simulink model "Diagrama de Dron NERV Protocol"  (R2026a)
settings: Solver=VariableStepAuto
undefined symbols (not defined in the file): A, adelante, antihorario, atras, bajar, boton1, boton2, boton3, boton4, boton5, camara, controladorm, derecha, encendido, G, gantihorario, ghorario, horario, izquierda, joystick1, joystick2, microcontrolador, modulowifi, S, subir, video

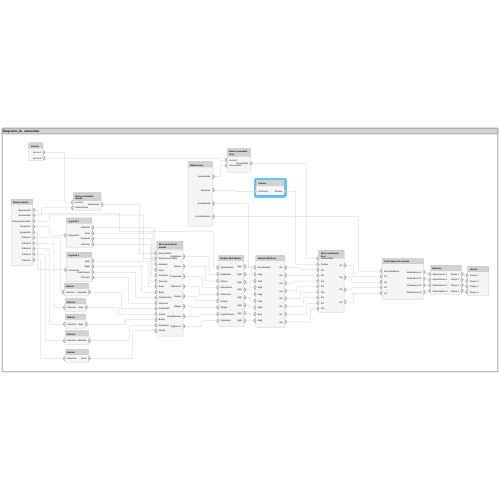
[thumbnail: Simulink's stored preview of the top-level diagram]
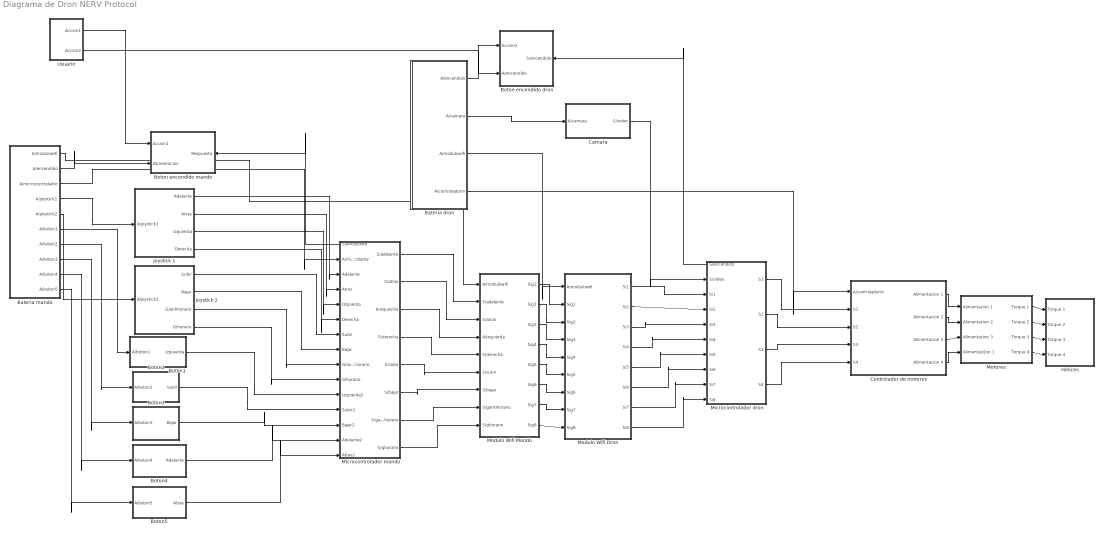
== system Diagrama de Dron NERV Protocol ==
  Bateria dron : Subsystem
      settings: PortSchema="{\"entries\":[{\"content\":{\"headerSize\":26,\"margin\":15,\"minimumSpacing\":25,\"sides\":[{\"content\":{},\"type\":\"ConnectorPlacement.EquallySpacedRectSide\",\"uuid\":\"2bf6d042-84ef-4730-88f6-3dff55cafecf\"},{\"content\":{\"connectorIds\":[\"Out1\",\"Out2\",\"Out3\",\"Out4\"],\"side\":\"RIGHT\"},\"type\":\"ConnectorPlacement.EquallySpacedRectSide\",\"uuid\":\"8f67bf94-d3d5-4da5-abec-0099f91d79d4\"},{\"content\":{\"side\":\"TOP\"},\"type\":\"ConnectorPlacement.EquallySpacedRectSide\",\"uuid\":\"7fdef67b-3e3b-4487-991c-040d13a0e676\"}]},\"type\":\"ConnectorPlacement.EquallySpacedConnector\",\"uuid\":\"d2ee6619-957d-4521-bbff-daa84c43e1b5\"}],\"packageUris\":[\"http://schema.mathworks.com/mf0/Connector/R2020b\"],\"version\":\"1.0\"}"
  Bateria mando : Subsystem
      settings: PortSchema="{\"entries\":[{\"content\":{\"headerSize\":26,\"margin\":15,\"minimumSpacing\":25,\"sides\":[{\"content\":{},\"type\":\"ConnectorPlacement.EquallySpacedRectSide\",\"uuid\":\"c8c9d0d9-9f51-4378-b4f1-417ae5560a64\"},{\"content\":{\"connectorIds\":[\"Out1\",\"Out2\",\"Out3\",\"Out4\",\"Out5\",\"Out6\",\"Out7\",\"Out8\",\"Out9\",\"Out10\"],\"side\":\"RIGHT\"},\"type\":\"ConnectorPlacement.EquallySpacedRectSide\",\"uuid\":\"af341b24-fdfa-4fbe-98c5-0f07d2be8a36\"},{\"content\":{\"side\":\"TOP\"},\"type\":\"ConnectorPlacement.EquallySpacedRectSide\",\"uuid\":\"c7c4f077-f713-4504-becb-cb3de254be2a\"}]},\"type\":\"ConnectorPlacement.EquallySpacedConnector\",\"uuid\":\"2a74e7c1-b664-434d-aa05-bb22f18d4dbf\"}],\"packageUris\":[\"http://schema.mathworks.com/mf0/Connector/R2020b\"],\"version\":\"1.0\"}"
  Boton encendido dron : Subsystem
      settings: PortSchema="{\"entries\":[{\"content\":{\"headerSize\":26,\"margin\":15,\"minimumSpacing\":25,\"sides\":[{\"content\":{\"connectorIds\":[\"In1\",\"In2\"]},\"type\":\"ConnectorPlacement.EquallySpacedRectSide\",\"uuid\":\"c8c9d0d9-9f51-4378-b4f1-417ae5560a64\"},{\"content\":{\"connectorIds\":[\"In3\"],\"side\":\"RIGHT\"},\"type\":\"ConnectorPlacement.EquallySpacedRectSide\",\"uuid\":\"af341b24-fdfa-4fbe-98c5-0f07d2be8a36\"},{\"content\":{\"side\":\"TOP\"},\"type\":\"ConnectorPlacement.EquallySpacedRectSide\",\"uuid\":\"c7c4f077-f713-4504-becb-cb3de254be2a\"}]},\"type\":\"ConnectorPlacement.EquallySpacedConnector\",\"uuid\":\"2a74e7c1-b664-434d-aa05-bb22f18d4dbf\"}],\"packageUris\":[\"http://schema.mathworks.com/mf0/Connector/R2020b\"],\"version\":\"1.0\"}"
  Boton encendido mando : Subsystem
      settings: PortSchema="{\"entries\":[{\"content\":{\"headerSize\":26,\"margin\":15,\"minimumSpacing\":25,\"sides\":[{\"content\":{\"connectorIds\":[\"In1\",\"In2\"]},\"type\":\"ConnectorPlacement.EquallySpacedRectSide\",\"uuid\":\"c8c9d0d9-9f51-4378-b4f1-417ae5560a64\"},{\"content\":{\"connectorIds\":[\"In3\"],\"side\":\"RIGHT\"},\"type\":\"ConnectorPlacement.EquallySpacedRectSide\",\"uuid\":\"af341b24-fdfa-4fbe-98c5-0f07d2be8a36\"},{\"content\":{\"side\":\"TOP\"},\"type\":\"ConnectorPlacement.EquallySpacedRectSide\",\"uuid\":\"c7c4f077-f713-4504-becb-cb3de254be2a\"}]},\"type\":\"ConnectorPlacement.EquallySpacedConnector\",\"uuid\":\"2a74e7c1-b664-434d-aa05-bb22f18d4dbf\"}],\"packageUris\":[\"http://schema.mathworks.com/mf0/Connector/R2020b\"],\"version\":\"1.0\"}"
  Boton1 : Subsystem
      settings: PortSchema="{\"entries\":[{\"content\":{\"headerSize\":26,\"margin\":15,\"minimumSpacing\":25,\"sides\":[{\"content\":{\"connectorIds\":[\"In1\"]},\"type\":\"ConnectorPlacement.EquallySpacedRectSide\",\"uuid\":\"859b65f9-1e56-49db-ad0e-625ee06f8163\"},{\"content\":{\"connectorIds\":[\"Out1\"],\"side\":\"RIGHT\"},\"type\":\"ConnectorPlacement.EquallySpacedRectSide\",\"uuid\":\"c49bccff-8b78-479d-ba62-905aef2a1b5e\"},{\"content\":{\"side\":\"TOP\"},\"type\":\"ConnectorPlacement.EquallySpacedRectSide\",\"uuid\":\"337def3d-9fc7-40b9-833c-a49097c9210f\"}]},\"type\":\"ConnectorPlacement.EquallySpacedConnector\",\"uuid\":\"a8accb01-4db9-4c00-8da7-dedce669f5d7\"}],\"packageUris\":[\"http://schema.mathworks.com/mf0/Connector/R2020b\"],\"version\":\"1.0\"}"
  Boton2 : Subsystem
      settings: PortSchema="{\"entries\":[{\"content\":{\"headerSize\":26,\"margin\":15,\"minimumSpacing\":25,\"sides\":[{\"content\":{\"connectorIds\":[\"In1\"]},\"type\":\"ConnectorPlacement.EquallySpacedRectSide\",\"uuid\":\"859b65f9-1e56-49db-ad0e-625ee06f8163\"},{\"content\":{\"connectorIds\":[\"Out1\"],\"side\":\"RIGHT\"},\"type\":\"ConnectorPlacement.EquallySpacedRectSide\",\"uuid\":\"c49bccff-8b78-479d-ba62-905aef2a1b5e\"},{\"content\":{\"side\":\"TOP\"},\"type\":\"ConnectorPlacement.EquallySpacedRectSide\",\"uuid\":\"337def3d-9fc7-40b9-833c-a49097c9210f\"}]},\"type\":\"ConnectorPlacement.EquallySpacedConnector\",\"uuid\":\"a8accb01-4db9-4c00-8da7-dedce669f5d7\"}],\"packageUris\":[\"http://schema.mathworks.com/mf0/Connector/R2020b\"],\"version\":\"1.0\"}"
  Boton3 : Subsystem
      settings: PortSchema="{\"entries\":[{\"content\":{\"headerSize\":26,\"margin\":15,\"minimumSpacing\":25,\"sides\":[{\"content\":{\"connectorIds\":[\"In1\"]},\"type\":\"ConnectorPlacement.EquallySpacedRectSide\",\"uuid\":\"859b65f9-1e56-49db-ad0e-625ee06f8163\"},{\"content\":{\"connectorIds\":[\"Out1\"],\"side\":\"RIGHT\"},\"type\":\"ConnectorPlacement.EquallySpacedRectSide\",\"uuid\":\"c49bccff-8b78-479d-ba62-905aef2a1b5e\"},{\"content\":{\"side\":\"TOP\"},\"type\":\"ConnectorPlacement.EquallySpacedRectSide\",\"uuid\":\"337def3d-9fc7-40b9-833c-a49097c9210f\"}]},\"type\":\"ConnectorPlacement.EquallySpacedConnector\",\"uuid\":\"a8accb01-4db9-4c00-8da7-dedce669f5d7\"}],\"packageUris\":[\"http://schema.mathworks.com/mf0/Connector/R2020b\"],\"version\":\"1.0\"}"
  Boton4 : Subsystem
      settings: PortSchema="{\"entries\":[{\"content\":{\"headerSize\":26,\"margin\":15,\"minimumSpacing\":25,\"sides\":[{\"content\":{\"connectorIds\":[\"In1\"]},\"type\":\"ConnectorPlacement.EquallySpacedRectSide\",\"uuid\":\"859b65f9-1e56-49db-ad0e-625ee06f8163\"},{\"content\":{\"connectorIds\":[\"Out1\"],\"side\":\"RIGHT\"},\"type\":\"ConnectorPlacement.EquallySpacedRectSide\",\"uuid\":\"c49bccff-8b78-479d-ba62-905aef2a1b5e\"},{\"content\":{\"side\":\"TOP\"},\"type\":\"ConnectorPlacement.EquallySpacedRectSide\",\"uuid\":\"337def3d-9fc7-40b9-833c-a49097c9210f\"}]},\"type\":\"ConnectorPlacement.EquallySpacedConnector\",\"uuid\":\"a8accb01-4db9-4c00-8da7-dedce669f5d7\"}],\"packageUris\":[\"http://schema.mathworks.com/mf0/Connector/R2020b\"],\"version\":\"1.0\"}"
  Boton5 : Subsystem
      settings: PortSchema="{\"entries\":[{\"content\":{\"headerSize\":26,\"margin\":15,\"minimumSpacing\":25,\"sides\":[{\"content\":{\"connectorIds\":[\"In1\"]},\"type\":\"ConnectorPlacement.EquallySpacedRectSide\",\"uuid\":\"859b65f9-1e56-49db-ad0e-625ee06f8163\"},{\"content\":{\"connectorIds\":[\"Out1\"],\"side\":\"RIGHT\"},\"type\":\"ConnectorPlacement.EquallySpacedRectSide\",\"uuid\":\"c49bccff-8b78-479d-ba62-905aef2a1b5e\"},{\"content\":{\"side\":\"TOP\"},\"type\":\"ConnectorPlacement.EquallySpacedRectSide\",\"uuid\":\"337def3d-9fc7-40b9-833c-a49097c9210f\"}]},\"type\":\"ConnectorPlacement.EquallySpacedConnector\",\"uuid\":\"a8accb01-4db9-4c00-8da7-dedce669f5d7\"}],\"packageUris\":[\"http://schema.mathworks.com/mf0/Connector/R2020b\"],\"version\":\"1.0\"}"
  Camara : Subsystem
      settings: PortSchema="{\"entries\":[{\"content\":{\"headerSize\":26,\"margin\":15,\"minimumSpacing\":25,\"sides\":[{\"content\":{\"connectorIds\":[\"In1\"]},\"type\":\"ConnectorPlacement.EquallySpacedRectSide\",\"uuid\":\"879727f6-324c-4f5e-9dc1-ac479d9c48af\"},{\"content\":{\"connectorIds\":[\"Out1\"],\"side\":\"RIGHT\"},\"type\":\"ConnectorPlacement.EquallySpacedRectSide\",\"uuid\":\"f3855134-d9a3-4d8c-bf73-dc4ed9d71427\"},{\"content\":{\"side\":\"TOP\"},\"type\":\"ConnectorPlacement.EquallySpacedRectSide\",\"uuid\":\"f26ad25d-e4a2-425b-a9d5-96d823958aa9\"}]},\"type\":\"ConnectorPlacement.EquallySpacedConnector\",\"uuid\":\"a98458b0-d022-4598-9285-5429fabca4b2\"}],\"packageUris\":[\"http://schema.mathworks.com/mf0/Connector/R2020b\"],\"version\":\"1.0\"}"
  Controlador de motores : Subsystem
      settings: PortSchema="{\"entries\":[{\"content\":{\"headerSize\":26,\"margin\":15,\"minimumSpacing\":25,\"sides\":[{\"content\":{\"connectorIds\":[\"In3\",\"In4\",\"In5\",\"In1\",\"In2\"]},\"type\":\"ConnectorPlacement.EquallySpacedRectSide\",\"uuid\":\"2bf6d042-84ef-4730-88f6-3dff55cafecf\"},{\"content\":{\"connectorIds\":[\"Out1\",\"Out2\",\"Out3\",\"Out4\"],\"side\":\"RIGHT\"},\"type\":\"ConnectorPlacement.EquallySpacedRectSide\",\"uuid\":\"8f67bf94-d3d5-4da5-abec-0099f91d79d4\"},{\"content\":{\"side\":\"TOP\"},\"type\":\"ConnectorPlacement.EquallySpacedRectSide\",\"uuid\":\"7fdef67b-3e3b-4487-991c-040d13a0e676\"},{\"content\":{\"side\":\"BOTTOM\"},\"type\":\"ConnectorPlacement.EquallySpacedRectSide\",\"uuid\":\"0c2c01ed-c52d-4b0b-a737-70a441f21ba4\"}]},\"type\":\"ConnectorPlacement.EquallySpacedConnector\",\"uuid\":\"d2ee6619-957d-4521-bbff-daa84c43e1b5\"}],\"packageUris\":[\"http://schema.mathworks.com/mf0/Connector/R2020b\"],\"version\":\"1.0\"}"
  Helices : Subsystem
      settings: PortSchema="{\"entries\":[{\"content\":{\"headerSize\":26,\"margin\":15,\"minimumSpacing\":25,\"sides\":[{\"content\":{\"connectorIds\":[\"In1\",\"In2\",\"In3\",\"In4\"]},\"type\":\"ConnectorPlacement.EquallySpacedRectSide\",\"uuid\":\"2bf6d042-84ef-4730-88f6-3dff55cafecf\"},{\"content\":{\"side\":\"RIGHT\"},\"type\":\"ConnectorPlacement.EquallySpacedRectSide\",\"uuid\":\"8f67bf94-d3d5-4da5-abec-0099f91d79d4\"},{\"content\":{\"side\":\"TOP\"},\"type\":\"ConnectorPlacement.EquallySpacedRectSide\",\"uuid\":\"7fdef67b-3e3b-4487-991c-040d13a0e676\"}]},\"type\":\"ConnectorPlacement.EquallySpacedConnector\",\"uuid\":\"d2ee6619-957d-4521-bbff-daa84c43e1b5\"}],\"packageUris\":[\"http://schema.mathworks.com/mf0/Connector/R2020b\"],\"version\":\"1.0\"}"
  Joystick 1 : Subsystem
      settings: PortSchema="{\"entries\":[{\"content\":{\"headerSize\":26,\"margin\":15,\"minimumSpacing\":25,\"sides\":[{\"content\":{\"connectorIds\":[\"In1\"]},\"type\":\"ConnectorPlacement.EquallySpacedRectSide\",\"uuid\":\"2bf6d042-84ef-4730-88f6-3dff55cafecf\"},{\"content\":{\"connectorIds\":[\"Out1\",\"Out2\",\"Out3\",\"Out4\"],\"side\":\"RIGHT\"},\"type\":\"ConnectorPlacement.EquallySpacedRectSide\",\"uuid\":\"8f67bf94-d3d5-4da5-abec-0099f91d79d4\"},{\"content\":{\"side\":\"TOP\"},\"type\":\"ConnectorPlacement.EquallySpacedRectSide\",\"uuid\":\"7fdef67b-3e3b-4487-991c-040d13a0e676\"}]},\"type\":\"ConnectorPlacement.EquallySpacedConnector\",\"uuid\":\"d2ee6619-957d-4521-bbff-daa84c43e1b5\"}],\"packageUris\":[\"http://schema.mathworks.com/mf0/Connector/R2020b\"],\"version\":\"1.0\"}"
  Joystick 2 : Subsystem
      settings: PortSchema="{\"entries\":[{\"content\":{\"headerSize\":26,\"margin\":15,\"minimumSpacing\":25,\"sides\":[{\"content\":{\"connectorIds\":[\"In1\"]},\"type\":\"ConnectorPlacement.EquallySpacedRectSide\",\"uuid\":\"2bf6d042-84ef-4730-88f6-3dff55cafecf\"},{\"content\":{\"connectorIds\":[\"Out1\",\"Out2\",\"Out3\",\"Out4\"],\"side\":\"RIGHT\"},\"type\":\"ConnectorPlacement.EquallySpacedRectSide\",\"uuid\":\"8f67bf94-d3d5-4da5-abec-0099f91d79d4\"},{\"content\":{\"side\":\"TOP\"},\"type\":\"ConnectorPlacement.EquallySpacedRectSide\",\"uuid\":\"7fdef67b-3e3b-4487-991c-040d13a0e676\"}]},\"type\":\"ConnectorPlacement.EquallySpacedConnector\",\"uuid\":\"d2ee6619-957d-4521-bbff-daa84c43e1b5\"}],\"packageUris\":[\"http://schema.mathworks.com/mf0/Connector/R2020b\"],\"version\":\"1.0\"}"
  Microcontrolador dron : Subsystem
      settings: PortSchema="{\"entries\":[{\"content\":{\"headerSize\":26,\"margin\":15,\"minimumSpacing\":25,\"sides\":[{\"content\":{\"connectorIds\":[\"Out5\",\"In1\",\"In2\",\"In3\",\"In4\",\"In5\",\"In6\",\"In7\",\"In8\",\"In9\"]},\"type\":\"ConnectorPlacement.EquallySpacedRectSide\",\"uuid\":\"859b65f9-1e56-49db-ad0e-625ee06f8163\"},{\"content\":{\"connectorIds\":[\"Out1\",\"Out2\",\"Out3\",\"Out4\"],\"side\":\"RIGHT\"},\"type\":\"ConnectorPlacement.EquallySpacedRectSide\",\"uuid\":\"c49bccff-8b78-479d-ba62-905aef2a1b5e\"},{\"content\":{\"side\":\"TOP\"},\"type\":\"ConnectorPlacement.EquallySpacedRectSide\",\"uuid\":\"337def3d-9fc7-40b9-833c-a49097c9210f\"}]},\"type\":\"ConnectorPlacement.EquallySpacedConnector\",\"uuid\":\"a8accb01-4db9-4c00-8da7-dedce669f5d7\"}],\"packageUris\":[\"http://schema.mathworks.com/mf0/Connector/R2020b\"],\"version\":\"1.0\"}"
  Microcontrolador mando : Subsystem
      settings: PortSchema="{\"entries\":[{\"content\":{\"headerSize\":26,\"margin\":15,\"minimumSpacing\":25,\"sides\":[{\"content\":{\"connectorIds\":[\"Out9\",\"In1\",\"In2\",\"In3\",\"In4\",\"In5\",\"In6\",\"In7\",\"In8\",\"In9\",\"In10\",\"In11\",\"In12\",\"In13\",\"In14\"]},\"type\":\"ConnectorPlacement.EquallySpacedRectSide\",\"uuid\":\"859b65f9-1e56-49db-ad0e-625ee06f8163\"},{\"content\":{\"connectorIds\":[\"Out1\",\"Out2\",\"Out3\",\"Out4\",\"Out5\",\"Out6\",\"Out7\",\"Out8\"],\"side\":\"RIGHT\"},\"type\":\"ConnectorPlacement.EquallySpacedRectSide\",\"uuid\":\"c49bccff-8b78-479d-ba62-905aef2a1b5e\"},{\"content\":{\"side\":\"TOP\"},\"type\":\"ConnectorPlacement.EquallySpacedRectSide\",\"uuid\":\"337def3d-9fc7-40b9-833c-a49097c9210f\"}]},\"type\":\"ConnectorPlacement.EquallySpacedConnector\",\"uuid\":\"a8accb01-4db9-4c00-8da7-dedce669f5d7\"}],\"packageUris\":[\"http://schema.mathworks.com/mf0/Connector/R2020b\"],\"version\":\"1.0\"}"
  Modulo Wifi Dron : Subsystem
      settings: PortSchema="{\"entries\":[{\"content\":{\"headerSize\":26,\"margin\":15,\"minimumSpacing\":25,\"sides\":[{\"content\":{\"connectorIds\":[\"In1\",\"In2\",\"In3\",\"In4\",\"In5\",\"In6\",\"In7\",\"In8\",\"In9\"]},\"type\":\"ConnectorPlacement.EquallySpacedRectSide\",\"uuid\":\"2bf6d042-84ef-4730-88f6-3dff55cafecf\"},{\"content\":{\"connectorIds\":[\"Out1\",\"Out2\",\"Out3\",\"Out4\",\"Out5\",\"Out6\",\"Out7\",\"Out8\"],\"side\":\"RIGHT\"},\"type\":\"ConnectorPlacement.EquallySpacedRectSide\",\"uuid\":\"8f67bf94-d3d5-4da5-abec-0099f91d79d4\"},{\"content\":{\"side\":\"TOP\"},\"type\":\"ConnectorPlacement.EquallySpacedRectSide\",\"uuid\":\"7fdef67b-3e3b-4487-991c-040d13a0e676\"}]},\"type\":\"ConnectorPlacement.EquallySpacedConnector\",\"uuid\":\"d2ee6619-957d-4521-bbff-daa84c43e1b5\"}],\"packageUris\":[\"http://schema.mathworks.com/mf0/Connector/R2020b\"],\"version\":\"1.0\"}"
  Modulo Wifi Mando : Subsystem
      settings: PortSchema="{\"entries\":[{\"content\":{\"headerSize\":26,\"margin\":15,\"minimumSpacing\":25,\"sides\":[{\"content\":{\"connectorIds\":[\"In1\",\"In2\",\"In3\",\"In4\",\"In5\",\"In6\",\"In7\",\"In8\",\"In9\"]},\"type\":\"ConnectorPlacement.EquallySpacedRectSide\",\"uuid\":\"2bf6d042-84ef-4730-88f6-3dff55cafecf\"},{\"content\":{\"connectorIds\":[\"Out1\",\"Out2\",\"Out3\",\"Out4\",\"Out5\",\"Out6\",\"Out7\",\"Out8\"],\"side\":\"RIGHT\"},\"type\":\"ConnectorPlacement.EquallySpacedRectSide\",\"uuid\":\"8f67bf94-d3d5-4da5-abec-0099f91d79d4\"},{\"content\":{\"side\":\"TOP\"},\"type\":\"ConnectorPlacement.EquallySpacedRectSide\",\"uuid\":\"7fdef67b-3e3b-4487-991c-040d13a0e676\"}]},\"type\":\"ConnectorPlacement.EquallySpacedConnector\",\"uuid\":\"d2ee6619-957d-4521-bbff-daa84c43e1b5\"}],\"packageUris\":[\"http://schema.mathworks.com/mf0/Connector/R2020b\"],\"version\":\"1.0\"}"
  Motores : Subsystem
      settings: PortSchema="{\"entries\":[{\"content\":{\"headerSize\":26,\"margin\":15,\"minimumSpacing\":25,\"sides\":[{\"content\":{\"connectorIds\":[\"In1\",\"In2\",\"In3\",\"In4\"]},\"type\":\"ConnectorPlacement.EquallySpacedRectSide\",\"uuid\":\"2bf6d042-84ef-4730-88f6-3dff55cafecf\"},{\"content\":{\"connectorIds\":[\"Out1\",\"Out2\",\"Out3\",\"Out4\"],\"side\":\"RIGHT\"},\"type\":\"ConnectorPlacement.EquallySpacedRectSide\",\"uuid\":\"8f67bf94-d3d5-4da5-abec-0099f91d79d4\"},{\"content\":{\"side\":\"TOP\"},\"type\":\"ConnectorPlacement.EquallySpacedRectSide\",\"uuid\":\"7fdef67b-3e3b-4487-991c-040d13a0e676\"}]},\"type\":\"ConnectorPlacement.EquallySpacedConnector\",\"uuid\":\"d2ee6619-957d-4521-bbff-daa84c43e1b5\"}],\"packageUris\":[\"http://schema.mathworks.com/mf0/Connector/R2020b\"],\"version\":\"1.0\"}"
  Usuario : Subsystem
      settings: PortSchema="{\"entries\":[{\"content\":{\"headerSize\":26,\"margin\":15,\"minimumSpacing\":25,\"sides\":[{\"content\":{},\"type\":\"ConnectorPlacement.EquallySpacedRectSide\",\"uuid\":\"c8c9d0d9-9f51-4378-b4f1-417ae5560a64\"},{\"content\":{\"connectorIds\":[\"Out1\",\"Out2\"],\"side\":\"RIGHT\"},\"type\":\"ConnectorPlacement.EquallySpacedRectSide\",\"uuid\":\"af341b24-fdfa-4fbe-98c5-0f07d2be8a36\"},{\"content\":{\"side\":\"TOP\"},\"type\":\"ConnectorPlacement.EquallySpacedRectSide\",\"uuid\":\"c7c4f077-f713-4504-becb-cb3de254be2a\"}]},\"type\":\"ConnectorPlacement.EquallySpacedConnector\",\"uuid\":\"2a74e7c1-b664-434d-aa05-bb22f18d4dbf\"}],\"packageUris\":[\"http://schema.mathworks.com/mf0/Connector/R2020b\"],\"version\":\"1.0\"}"
  wires:
  Motores/4(Torque 4) -> Helices/4(Torque 4)
  Motores/3(Torque 3) -> Helices/3(Torque 3)
  Motores/2(Torque 2) -> Helices/2(Torque 2)
  Motores/1(Torque 1) -> Helices/1(Torque 1)
  Controlador de motores/4(Alimentacion 4) -> Motores/4(Alimentaci[on 1)
  Controlador de motores/3(Alimentacion 3) -> Motores/3(Alimentacion 3)
  Controlador de motores/2(Alimentacion 2) -> Motores/2(Alimentacion 2)
  Controlador de motores/1(Alimentacion 1) -> Motores/1(Alimentacion 1)
  Modulo Wifi Mando/1(Sig1) -> Modulo Wifi Dron/2(Sig1)
  Modulo Wifi Mando/2(Sig2) -> Modulo Wifi Dron/3(Sig2)
  Modulo Wifi Mando/3(Sig3) -> Modulo Wifi Dron/4(Sig3)
  Modulo Wifi Mando/4(Sig4) -> Modulo Wifi Dron/5(Sig4)
  Bateria mando/2(A/encendido) -> Boton encendido mando/2(Alimentacion)
  Usuario/1(Accion1) -> Boton encendido mando/1(Accion1)
  Usuario/2(Accion2) -> Boton encendido dron/1(Accion2)
  Bateria dron/1(A/encendido) -> Boton encendido dron/2(A/encendido)
  Microcontrolador mando/9(S/encendido) -> Boton encendido mando/3(Respuesta)
  Bateria mando/3(A/microcontrolador) -> Microcontrolador mando/1(A/microcontrolador)
  Bateria mando/4(A/joystick1) -> Joystick 1/1(A/joystick1)
  Bateria mando/5(A/joystick2) -> Joystick 2/1(A/joystick2)
  Bateria mando/6(A/boton1) -> Boton1/1(A/boton1)
  Bateria mando/7(A/boton2) -> Boton2/1(A/boton2)
  Bateria mando/8(A/boton3) -> Boton3/1(A/boton3)
  Bateria mando/9(A/boton4) -> Boton4/1(A/boton4)
  Bateria mando/10(A/boton5) -> Boton5/1(A/boton5)
  Joystick 1/1(Adelante) -> Microcontrolador mando/2(Adelante)
  Joystick 1/2(Atras) -> Microcontrolador mando/3(Atras)
  Joystick 1/3(Izquierda) -> Microcontrolador mando/4(Izquierda)
  Joystick 1/4(Derecha) -> Microcontrolador mando/5(Derecha)
  Joystick 2/1(Subir) -> Microcontrolador mando/6(Subir)
  Joystick 2/2(Bajar) -> Microcontrolador mando/7(Bajar)
  Joystick 2/3(G/antihorario) -> Microcontrolador mando/8(G/antihorario)
  Joystick 2/4(G/horario) -> Microcontrolador mando/9(G/horario)
  Boton1/1(Izquierda) -> Microcontrolador mando/10(Izquierda2)
  Boton2/1(Subir) -> Microcontrolador mando/11(Subir2)
  Boton3/1(Bajar) -> Microcontrolador mando/12(Bajar2)
  Boton4/1(Adelante) -> Microcontrolador mando/13(Adelante2)
  Boton5/1(Atras) -> Microcontrolador mando/14(Atras2)
  Microcontrolador dron/5(S/encendido) -> Boton encendido dron/3(S/encendido)
  Bateria mando/1(A/modulowifi) -> Modulo Wifi Mando/1(A/modulowifi)
  Bateria dron/3(A/modulowifi) -> Modulo Wifi Dron/1(A/modulowifi)
  Bateria dron/4(A/controladorm) -> Controlador de motores/3(A/controladorm)
  Microcontrolador dron/1(S1) -> Controlador de motores/4(S1)
  Microcontrolador dron/2(S2) -> Controlador de motores/5(S2)
  Microcontrolador dron/3(S3) -> Controlador de motores/1(S3)
  Microcontrolador dron/4(S4) -> Controlador de motores/2(S4)
  Microcontrolador mando/1(S/adelante) -> Modulo Wifi Mando/2(S/adelante)
  Microcontrolador mando/2(S/atras) -> Modulo Wifi Mando/3(S/atras)
  Microcontrolador mando/3(A/izquierda) -> Modulo Wifi Mando/4(A/izquierda)
  Microcontrolador mando/4(S/derecha) -> Modulo Wifi Mando/5(S/derecha)
  Microcontrolador mando/5(S/subir) -> Modulo Wifi Mando/6(S/subir)
  Microcontrolador mando/6(S/bajar) -> Modulo Wifi Mando/7(S/bajar)
  Microcontrolador mando/7(S/gantihorario) -> Modulo Wifi Mando/8(S/gantihorario)
  Microcontrolador mando/8(S/ghorario) -> Modulo Wifi Mando/9(S/ghorario)
  Modulo Wifi Mando/5(Sig5) -> Modulo Wifi Dron/6(Sig5)
  Modulo Wifi Mando/6(Sig6) -> Modulo Wifi Dron/7(Sig6)
  Modulo Wifi Mando/7(Sig7) -> Modulo Wifi Dron/8(Sig7)
  Modulo Wifi Mando/8(Sig8) -> Modulo Wifi Dron/9(Sig8)
  Modulo Wifi Dron/1(Si1) -> Microcontrolador dron/2(Si1)
  Modulo Wifi Dron/2(Si2) -> Microcontrolador dron/3(Si2)
  Modulo Wifi Dron/3(Si3) -> Microcontrolador dron/4(Si3)
  Modulo Wifi Dron/4(Si4) -> Microcontrolador dron/5(Si4)
  Modulo Wifi Dron/5(Si5) -> Microcontrolador dron/6(Si5)
  Modulo Wifi Dron/6(Si6) -> Microcontrolador dron/7(Si6)
  Modulo Wifi Dron/7(Si7) -> Microcontrolador dron/8(Si7)
  Modulo Wifi Dron/8(Si8) -> Microcontrolador dron/9(Si8)
  Bateria dron/2(A/camara) -> Camara/1(A/camara)
  Camara/1(S/video) -> Microcontrolador dron/1(S/video)

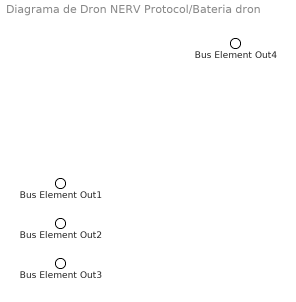
== system Diagrama de Dron NERV Protocol/Bateria dron ==
  Bus Element Out1 : Outport  PortName=A/encendido
  Bus Element Out4 : Outport  Port=2  PortName=A/camara
  Bus Element Out2 : Outport  Port=3  PortName=A/modulowifi
  Bus Element Out3 : Outport  Port=4  PortName=A/controladorm

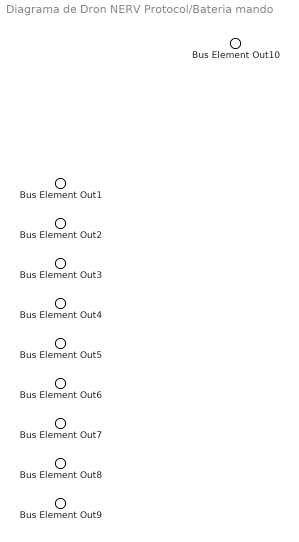
== system Diagrama de Dron NERV Protocol/Bateria mando ==
  Bus Element Out10 : Outport  PortName=A/modulowifi
  Bus Element Out1 : Outport  Port=2  PortName=A/encendido
  Bus Element Out2 : Outport  Port=3  PortName=A/microcontrolador
  Bus Element Out3 : Outport  Port=4  PortName=A/joystick1
  Bus Element Out4 : Outport  Port=5  PortName=A/joystick2
  Bus Element Out5 : Outport  Port=6  PortName=A/boton1
  Bus Element Out6 : Outport  Port=7  PortName=A/boton2
  Bus Element Out7 : Outport  Port=8  PortName=A/boton3
  Bus Element Out8 : Outport  Port=9  PortName=A/boton4
  Bus Element Out9 : Outport  Port=10  PortName=A/boton5

== system Diagrama de Dron NERV Protocol/Boton encendido dron ==
  Bus Element In3 : Inport  PortName=Accion2
  Bus Element In2 : Inport  Port=2  PortName=A/encendido
  Bus Element In1 : Inport  Port=3  PortName=S/encendido

== system Diagrama de Dron NERV Protocol/Boton encendido mando ==
  Bus Element In3 : Inport  PortName=Accion1
  Bus Element In2 : Inport  Port=2  PortName=Alimentacion
  Bus Element In1 : Inport  Port=3  PortName=Respuesta

== system Diagrama de Dron NERV Protocol/Boton1 ==
  Bus Element In1 : Inport  PortName=A/boton1
  Bus Element Out1 : Outport  PortName=Izquierda

== system Diagrama de Dron NERV Protocol/Boton2 ==
  Bus Element In1 : Inport  PortName=A/boton2
  Bus Element Out1 : Outport  PortName=Subir

== system Diagrama de Dron NERV Protocol/Boton3 ==
  Bus Element In1 : Inport  PortName=A/boton3
  Bus Element Out1 : Outport  PortName=Bajar

== system Diagrama de Dron NERV Protocol/Boton4 ==
  Bus Element In1 : Inport  PortName=A/boton4
  Bus Element Out1 : Outport  PortName=Adelante

== system Diagrama de Dron NERV Protocol/Boton5 ==
  Bus Element In1 : Inport  PortName=A/boton5
  Bus Element Out1 : Outport  PortName=Atras

== system Diagrama de Dron NERV Protocol/Camara ==
  Bus Element In1 : Inport  PortName=A/camara
  Bus Element Out1 : Outport  PortName=S/video

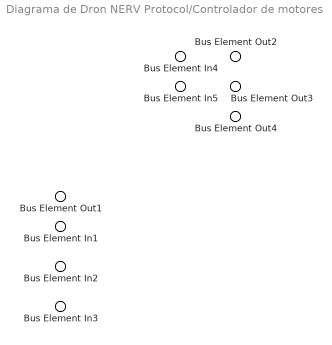
== system Diagrama de Dron NERV Protocol/Controlador de motores ==
  Bus Element In4 : Inport  PortName=S3
  Bus Element In5 : Inport  Port=2  PortName=S4
  Bus Element In1 : Inport  Port=3  PortName=A/controladorm
  Bus Element In2 : Inport  Port=4  PortName=S1
  Bus Element In3 : Inport  Port=5  PortName=S2
  Bus Element Out4 : Outport  PortName=Alimentacion 1
  Bus Element Out3 : Outport  Port=2  PortName=Alimentacion 2
  Bus Element Out2 : Outport  Port=3  PortName=Alimentacion 3
  Bus Element Out1 : Outport  Port=4  PortName=Alimentacion 4

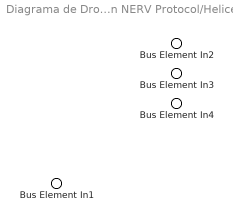
== system Diagrama de Dron NERV Protocol/Helices ==
  Bus Element In4 : Inport  PortName=Torque 1
  Bus Element In3 : Inport  Port=2  PortName=Torque 2
  Bus Element In2 : Inport  Port=3  PortName=Torque 3
  Bus Element In1 : Inport  Port=4  PortName=Torque 4

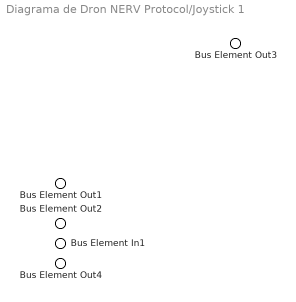
== system Diagrama de Dron NERV Protocol/Joystick 1 ==
  Bus Element In1 : Inport  PortName=A/joystick1
  Bus Element Out1 : Outport  PortName=Adelante
  Bus Element Out3 : Outport  Port=2  PortName=Atras
  Bus Element Out2 : Outport  Port=3  PortName=Izquierda
  Bus Element Out4 : Outport  Port=4  PortName=Derecha

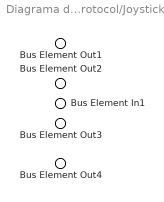
== system Diagrama de Dron NERV Protocol/Joystick 2 ==
  Bus Element In1 : Inport  PortName=A/joystick2
  Bus Element Out1 : Outport  PortName=Subir
  Bus Element Out2 : Outport  Port=2  PortName=Bajar
  Bus Element Out3 : Outport  Port=3  PortName=G/antihorario
  Bus Element Out4 : Outport  Port=4  PortName=G/horario

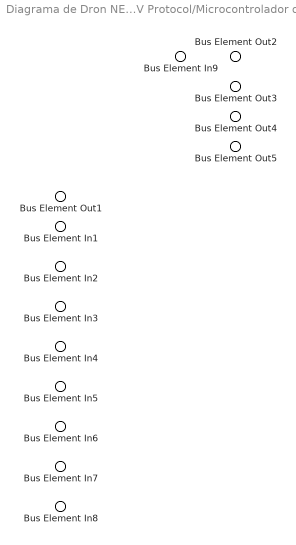
== system Diagrama de Dron NERV Protocol/Microcontrolador dron ==
  Bus Element In9 : Inport  PortName=S/video
  Bus Element In1 : Inport  Port=2  PortName=Si1
  Bus Element In2 : Inport  Port=3  PortName=Si2
  Bus Element In3 : Inport  Port=4  PortName=Si3
  Bus Element In4 : Inport  Port=5  PortName=Si4
  Bus Element In5 : Inport  Port=6  PortName=Si5
  Bus Element In6 : Inport  Port=7  PortName=Si6
  Bus Element In7 : Inport  Port=8  PortName=Si7
  Bus Element In8 : Inport  Port=9  PortName=Si8
  Bus Element Out2 : Outport  PortName=S1
  Bus Element Out3 : Outport  Port=2  PortName=S2
  Bus Element Out4 : Outport  Port=3  PortName=S3
  Bus Element Out5 : Outport  Port=4  PortName=S4
  Bus Element Out1 : Outport  Port=5  PortName=S/encendido

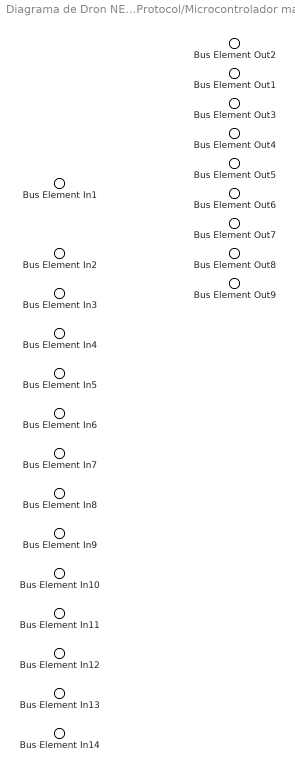
== system Diagrama de Dron NERV Protocol/Microcontrolador mando ==
  Bus Element In1 : Inport  PortName=A/microcontrolador
  Bus Element In2 : Inport  Port=2  PortName=Adelante
  Bus Element In3 : Inport  Port=3  PortName=Atras
  Bus Element In4 : Inport  Port=4  PortName=Izquierda
  Bus Element In5 : Inport  Port=5  PortName=Derecha
  Bus Element In6 : Inport  Port=6  PortName=Subir
  Bus Element In7 : Inport  Port=7  PortName=Bajar
  Bus Element In8 : Inport  Port=8  PortName=G/antihorario
  Bus Element In9 : Inport  Port=9  PortName=G/horario
  Bus Element In10 : Inport  Port=10  PortName=Izquierda2
  Bus Element In11 : Inport  Port=11  PortName=Subir2
  Bus Element In12 : Inport  Port=12  PortName=Bajar2
  Bus Element In13 : Inport  Port=13  PortName=Adelante2
  Bus Element In14 : Inport  Port=14  PortName=Atras2
  Bus Element Out1 : Outport  PortName=S/adelante
  Bus Element Out3 : Outport  Port=2  PortName=S/atras
  Bus Element Out4 : Outport  Port=3  PortName=A/izquierda
  Bus Element Out5 : Outport  Port=4  PortName=S/derecha
  Bus Element Out6 : Outport  Port=5  PortName=S/subir
  Bus Element Out7 : Outport  Port=6  PortName=S/bajar
  Bus Element Out8 : Outport  Port=7  PortName=S/gantihorario
  Bus Element Out9 : Outport  Port=8  PortName=S/ghorario
  Bus Element Out2 : Outport  Port=9  PortName=S/encendido

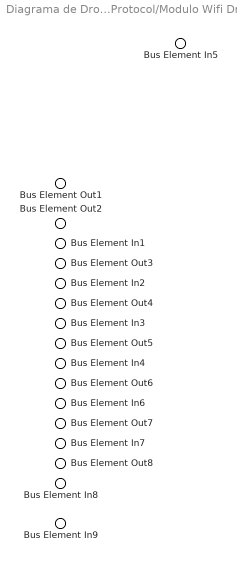
== system Diagrama de Dron NERV Protocol/Modulo Wifi Dron ==
  Bus Element In5 : Inport  PortName=A/modulowifi
  Bus Element In1 : Inport  Port=2  PortName=Sig1
  Bus Element In2 : Inport  Port=3  PortName=Sig2
  Bus Element In3 : Inport  Port=4  PortName=Sig3
  Bus Element In4 : Inport  Port=5  PortName=Sig4
  Bus Element In6 : Inport  Port=6  PortName=Sig5
  Bus Element In7 : Inport  Port=7  PortName=Sig6
  Bus Element In8 : Inport  Port=8  PortName=Sig7
  Bus Element In9 : Inport  Port=9  PortName=Sig8
  Bus Element Out1 : Outport  PortName=Si1
  Bus Element Out2 : Outport  Port=2  PortName=Si2
  Bus Element Out3 : Outport  Port=3  PortName=Si3
  Bus Element Out4 : Outport  Port=4  PortName=Si4
  Bus Element Out5 : Outport  Port=5  PortName=Si5
  Bus Element Out6 : Outport  Port=6  PortName=Si6
  Bus Element Out7 : Outport  Port=7  PortName=Si7
  Bus Element Out8 : Outport  Port=8  PortName=Si8

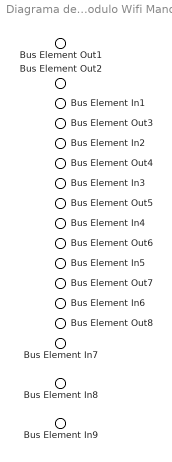
== system Diagrama de Dron NERV Protocol/Modulo Wifi Mando ==
  Bus Element In1 : Inport  PortName=A/modulowifi
  Bus Element In2 : Inport  Port=2  PortName=S/adelante
  Bus Element In3 : Inport  Port=3  PortName=S/atras
  Bus Element In4 : Inport  Port=4  PortName=A/izquierda
  Bus Element In5 : Inport  Port=5  PortName=S/derecha
  Bus Element In6 : Inport  Port=6  PortName=S/subir
  Bus Element In7 : Inport  Port=7  PortName=S/bajar
  Bus Element In8 : Inport  Port=8  PortName=S/gantihorario
  Bus Element In9 : Inport  Port=9  PortName=S/ghorario
  Bus Element Out1 : Outport  PortName=Sig1
  Bus Element Out2 : Outport  Port=2  PortName=Sig2
  Bus Element Out3 : Outport  Port=3  PortName=Sig3
  Bus Element Out4 : Outport  Port=4  PortName=Sig4
  Bus Element Out5 : Outport  Port=5  PortName=Sig5
  Bus Element Out6 : Outport  Port=6  PortName=Sig6
  Bus Element Out7 : Outport  Port=7  PortName=Sig7
  Bus Element Out8 : Outport  Port=8  PortName=Sig8

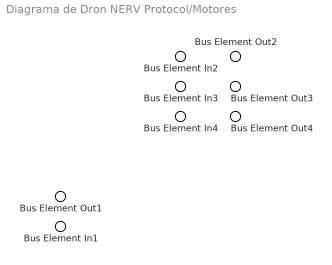
== system Diagrama de Dron NERV Protocol/Motores ==
  Bus Element In4 : Inport  PortName=Alimentacion 1
  Bus Element In3 : Inport  Port=2  PortName=Alimentacion 2
  Bus Element In2 : Inport  Port=3  PortName=Alimentacion 3
  Bus Element In1 : Inport  Port=4  PortName=Alimentaci[on 1
  Bus Element Out4 : Outport  PortName=Torque 1
  Bus Element Out3 : Outport  Port=2  PortName=Torque 2
  Bus Element Out2 : Outport  Port=3  PortName=Torque 3
  Bus Element Out1 : Outport  Port=4  PortName=Torque 4

== system Diagrama de Dron NERV Protocol/Usuario ==
  Bus Element Out1 : Outport  PortName=Accion1
  Bus Element Out2 : Outport  Port=2  PortName=Accion2
